simulink model "MRAC_Plant"  (R2021a)
settings: Solver=ode45  StartTime=0.0  StopTime=300  MaxStep=0.2  RelTol=1e-5
settings Model: Creator=Denilson Nicolau  LastModifiedBy=Denilson Nicolau

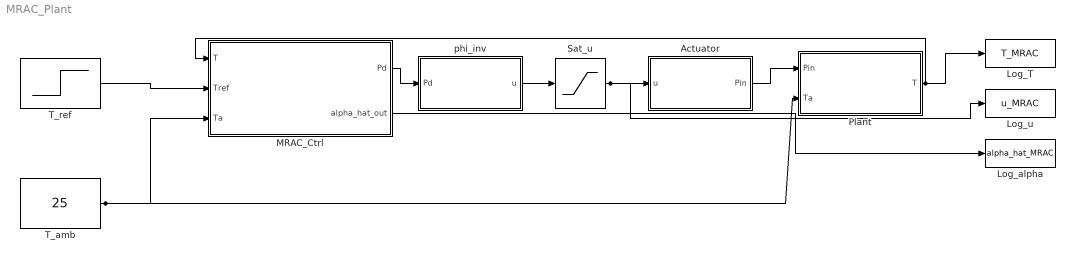
== system MRAC_Plant ==
  Actuator : MATLAB Function  TreatAsAtomicUnit=on
  Log_T : ToWorkspace  VariableName=T_MRAC  SaveFormat=Timeseries  SampleTime=-1
  Log_alpha : ToWorkspace  VariableName=alpha_hat_MRAC  SaveFormat=Timeseries  SampleTime=-1
  Log_u : ToWorkspace  VariableName=u_MRAC  SaveFormat=Timeseries  SampleTime=-1
  MRAC_Ctrl : Subsystem
  Plant : Subsystem
  Sat_u : Saturate  UpperLimit=1.057  LowerLimit=0
  T_amb : Constant  Value=25
  T_ref : Step  Time=0  Before=25  After=70  SampleTime=0
  phi_inv : MATLAB Function  TreatAsAtomicUnit=on
  wires:
  Plant/1(T) -> MRAC_Ctrl/1(T), Log_T/1
  T_ref/1 -> MRAC_Ctrl/2(Tref)
  T_amb/1 -> MRAC_Ctrl/3(Ta), Plant/2(Ta)
  MRAC_Ctrl/1(Pd) -> phi_inv/1(Pd)
  phi_inv/1(u) -> Sat_u/1
  Sat_u/1 -> Actuator/1(u), Log_u/1
  Actuator/1(Pin) -> Plant/1(Pin)
  MRAC_Ctrl/2(alpha_hat_out) -> Log_alpha/1

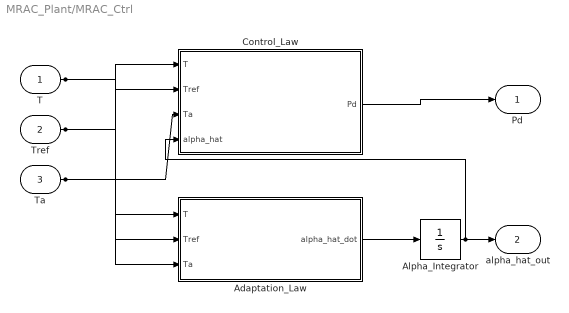
== system MRAC_Plant/MRAC_Ctrl ==
  T : Inport
  Tref : Inport  Port=2
  Ta : Inport  Port=3
  Adaptation_Law : MATLAB Function  TreatAsAtomicUnit=on
  Alpha_Integrator : Integrator  InitialCondition=0.0167
  Control_Law : MATLAB Function  TreatAsAtomicUnit=on
  Pd : Outport
  alpha_hat_out : Outport  Port=2
  wires:
  T/1 -> Control_Law/1(T), Adaptation_Law/1(T)
  Tref/1 -> Control_Law/2(Tref), Adaptation_Law/2(Tref)
  Ta/1 -> Control_Law/3(Ta), Adaptation_Law/3(Ta)
  Adaptation_Law/1(alpha_hat_dot) -> Alpha_Integrator/1
  Alpha_Integrator/1 -> Control_Law/4(alpha_hat), alpha_hat_out/1
  Control_Law/1(Pd) -> Pd/1

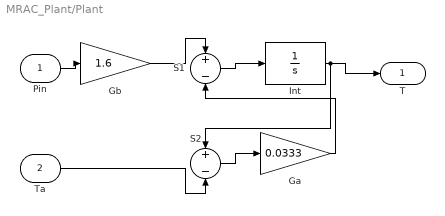
== system MRAC_Plant/Plant ==
  Pin : Inport
  Ta : Inport  Port=2
  Ga : Gain  Gain=0.0333
  Gb : Gain  Gain=1.6
  Int : Integrator  InitialCondition=25
  S1 : Sum  Inputs=+-
  S2 : Sum  Inputs=+-
  T : Outport
  wires:
  Pin/1 -> Gb/1
  Gb/1 -> S1/1
  Ga/1 -> S1/2
  S1/1 -> Int/1
  Int/1 -> T/1, S2/1
  Ta/1 -> S2/2
  S2/1 -> Ga/1

== matlab function MRAC_Plant/Actuator ==
  data: u input; Pin output
function Pin = Actuator(u)
%%#codegen
  Pin = (10^(4*double(u) - 1)) / 200;
end

== matlab function MRAC_Plant/phi_inv ==
  data: Pd input; u output
function u = phi_inv(Pd)
%%#codegen
  Pd = max(1e-6, min(2.42, double(Pd)));
  u  = (log10(200*Pd) + 1) / 4;
end

== matlab function MRAC_Plant/MRAC_Ctrl/Control_Law ==
  data: T input; Pd output; Tref input; Ta input; alpha_hat input
function Pd = Control_Law(T, Tref, Ta, alpha_hat)
%#codegen
  beta  = 1.6;
  k_a   = 1.2;
  P_max = 2.42;
  e = double(T) - double(Tref);
  W = double(T) - double(Ta);
  Pd = (1/beta) * (alpha_hat * W - k_a * e);
  Pd = max(0, min(P_max, Pd));
end

== matlab function MRAC_Plant/MRAC_Ctrl/Adaptation_Law ==
  data: T input; alpha_hat_dot output; Tref input; Ta input
function alpha_hat_dot = Adaptation_Law(T, Tref, Ta)
%#codegen
  gamma = 5e-05;
  e = double(T) - double(Tref);
  W = double(T) - double(Ta);
  alpha_hat_dot = -gamma * e * W;
end
